simulink model "testmodel_1109"  (R2015b)
settings: Solver=FixedStepDiscrete  StartTime=0.0  StopTime=50  FixedStep=Ts  RelTol=1e-3
PreLoadFcn:
  | Ts_IO601 = 0.001;
InitFcn:
  | Ts_IO601 = 0.001;
  | Ts=0.004;
libraries: canmsglib x14, speedgoatlib_IO601 x9, slrtlib x9, simulink x3
settings Model: Creator=lab2  LastModifiedBy=1SMARTe
settings SolverCC: EnableConcurrentExecution=on
settings DataIOCC: SaveFormat=Array
settings OptimizationCC: BlockReduction=off  OptimizeBlockIOStorage=off  BufferReuse=off  GlobalBufferReuse=off  ExpressionFolding=off  LocalBlockOutputs=off
settings DebuggingCC: UnconnectedInputMsg=none  UnconnectedOutputMsg=none  UnconnectedLineMsg=none
settings HardwareCC: ProdBitPerPointer=32  ProdLargestAtomicFloat=None  ProdWordSize=32  ProdLongLongMode=on  ProdHWDeviceType=Generic->32-bit x86 compatible
settings RTWCC: SystemTargetFile=slrt.tlc  TemplateMakefile=slrt_default_tmf  Description=Simulink Real-Time  RTWCompilerOptimization=on
settings ConfigComp: CovModelRefEnable=Off

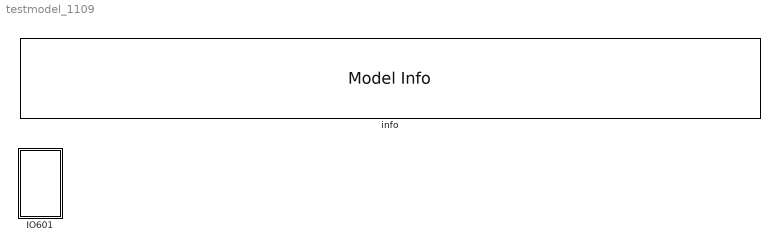
== system testmodel_1109 ==
  IO601 : Subsystem
  info : simulink/Model-Wide Utilities/Model Info  Frame=on  DisplayStringWithTags=|  HorizontalTextAlignment=Left  LeftAlignmentValue=0.02  SourceBlockDiagram=testmodel_1109  TagMaxNumber=20
      | SPEEDGOAT Simulink Real-Time  test model for Real-time target machine (SN2820)
      | prepared by Speedgoat with MATLAB R2015a
      | 
      | Build date: %<Created>

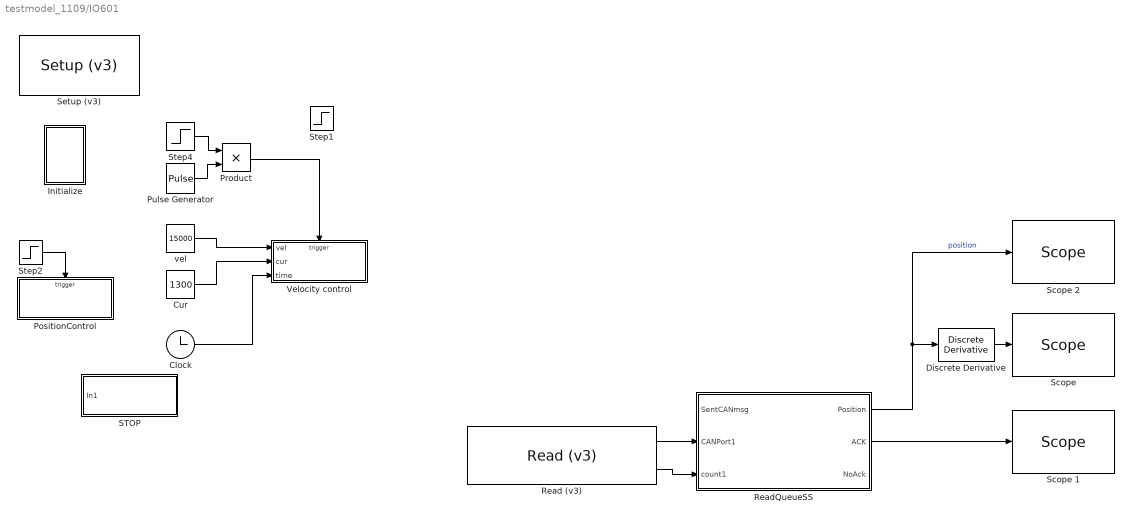
== system testmodel_1109/IO601 ==
  Clock : Clock
  Cur : Constant  Value=1300  OutMin=1100  OutMax=1500  OutDataTypeStr=uint32
  Discrete Derivative : simulink/Discrete/Discrete Derivative  gainval=1.0  ICPrevScaledInput=0.0  InputProcessing=Inherited  OutMin=[]  OutMax=[]  OutDataType=fixdt(1, 16)  OutScaling=2^-10  DoSatur=off
  Initialize : Subsystem
  "PositionControl " : Subsystem  TreatAsAtomicUnit=on
  Product : Product
  Pulse Generator : DiscretePulseGenerator  PulseType=Time based  Period=Ts*10  PulseWidth=10  PhaseDelay=10  SampleTime=Ts_IO601
  Read (v3) : speedgoatlib_IO601/Read (v3)  id=1  outputFormat=Vector of CAN_MESSAGE  port1=on  port2=off  depth1=37  depth2=4  sampletime=Ts  pciSlot=-1
  ReadQueueSS : Subsystem
  STOP : Subsystem  TreatAsAtomicUnit=on
  "Scope " : slrtlib/Displays and Logging/Scope   scopeno=3  scopetype=Target  autostart=on  viewmode=Graphical sliding  formatstr='%15.6f'  grid=on  ylimits=[0000,0000]  nosamples=50/Ts  noprepostsamples=0  interleave=1  triggermode=FreeRun  triggersignal=1  trigsignalfromport=off  triggerlevel=0.0  triggerslope=Either  triggerscope=1  triggersample=0  filename=data.dat  mode=Lazy  writesize=512  autorestart=off  dynamicfilemode=off  maxwritefilesize=512*1024^2
  Scope 1 : slrtlib/Displays and Logging/Scope   scopeno=12  scopetype=Target  autostart=on  viewmode=Numerical  formatstr='%15.6f'  grid=on  ylimits=[0000,0000]  nosamples=50/Ts  noprepostsamples=0  interleave=1  triggermode=FreeRun  triggersignal=1  trigsignalfromport=on  triggerlevel=0.0  triggerslope=Either  triggerscope=1  triggersample=0  filename=data.dat  mode=Lazy  writesize=512  autorestart=off  dynamicfilemode=off  maxwritefilesize=512*1024^2
  Scope 2 : slrtlib/Displays and Logging/Scope   scopeno=2  scopetype=Target  autostart=on  viewmode=Graphical sliding  formatstr='%15.6f'  grid=on  ylimits=[0000,0000]  nosamples=50/Ts  noprepostsamples=0  interleave=1  triggermode=FreeRun  triggersignal=1  trigsignalfromport=off  triggerlevel=0.0  triggerslope=Either  triggerscope=1  triggersample=0  filename=data.dat  mode=Lazy  writesize=512  autorestart=off  dynamicfilemode=off  maxwritefilesize=512*1024^2
  Setup (v3) : speedgoatlib_IO601/Setup (v3)  id=1  can1enable=on  can1bus=Highspeed  can1Baudrate=1 MBaud  can1UserBR=[1,1,5,2]  stdAcc1=[0,0,0,0]  extAcc1=[0,0,0,0]  can2enable=on  can2bus=Highspeed  can2Baudrate=1 MBaud  can2UserBR=[1,1,5,2]  stdAcc2=[0,0,0,0]  extAcc2=[0,0,0,0]  pciSlot=-1
  Step1 : Step  Time=10  SampleTime=Ts
  Step2 : Step  Time=25  SampleTime=Ts
  Step4 : Step  Time=14  Before=1  After=0  SampleTime=0
  Velocity control : Subsystem  TreatAsAtomicUnit=on
  "vel " : Constant  Value=15000  OutMin=0  OutMax=20000  OutDataTypeStr=uint32
  wires:
  Step4/1 -> Product/1
  Pulse Generator/1 -> Product/2
  ReadQueueSS/2(ACK) -> Scope 1/1
  Cur/1 -> Velocity control/2(cur)
  "vel "/1 -> Velocity control/1(vel)
  ReadQueueSS/1(Position) -> Discrete Derivative/1, Scope 2/1  "position"
  Discrete Derivative/1 -> "Scope "/1
  Read (v3)/1 -> ReadQueueSS/2(CANPort1)
  Read (v3)/2 -> ReadQueueSS/3(count1)
  Step2/1 -> "PositionControl "/Trigger
  Product/1 -> Velocity control/Trigger
  Clock/1 -> Velocity control/3(time)

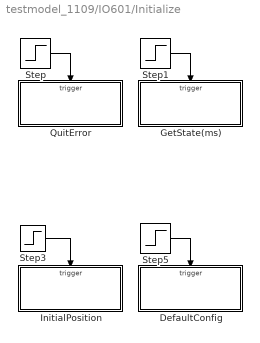
== system testmodel_1109/IO601/Initialize ==
  DefaultConfig : Subsystem  TreatAsAtomicUnit=on
  GetState(ms) : Subsystem  TreatAsAtomicUnit=on
  InitialPosition : Subsystem  TreatAsAtomicUnit=on
  QuitError : Subsystem  TreatAsAtomicUnit=on
  Step : Step  SampleTime=Ts
  Step1 : Step  Time=2  SampleTime=Ts
  Step3 : Step  Time=2  SampleTime=Ts
  Step5 : Step  Time=15  SampleTime=Ts
  wires:
  Step/1 -> QuitError/Trigger
  Step3/1 -> InitialPosition/Trigger
  Step5/1 -> DefaultConfig/Trigger
  Step1/1 -> GetState(ms)/Trigger

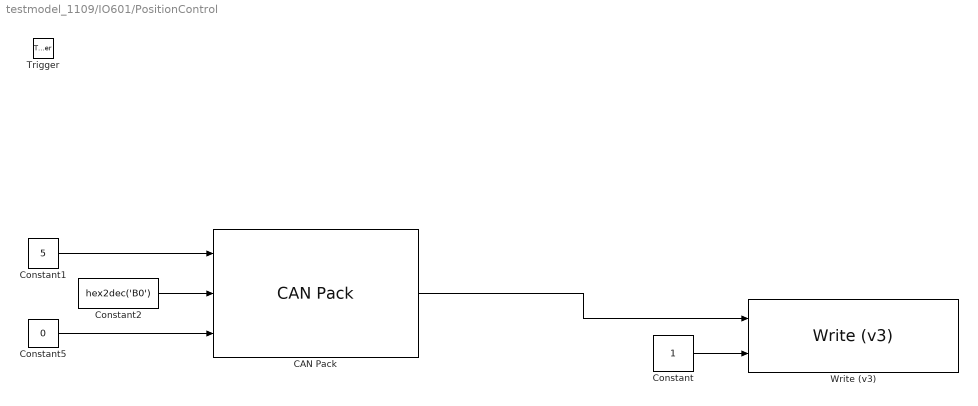
== system testmodel_1109/IO601/PositionControl  ==
  Trigger : TriggerPort
  CAN Pack : canmsglib/CAN Pack  MsgList=(none)  MsgName=Position Msg  MsgIDType=Standard (11-bit identifier)  MsgIdentifier=hex2dec('503')  MsgLength=6  SignalInfo=Signal1$0$8$1$2$1$0$1$0$-Inf$Inf$#Signal2$8$8$1$2$1$0$1$0$-Inf$Inf$#Signal3$16$32$1$1$1$0$1$0$-Inf$Inf$#  NSignals=3  StartBits=str2num('[int32(0);int32(8);int32(16)]')  SignalSizes=str2num('[int32(8);int32(8);int32(32)]')  ByteOrders=str2num('[int32(1);int32(1);int32(1)]')  DataTypes=str2num('[int32(2);int32(2);int32(1)]')  MultiplexTypes=str2num('[int32(1);int32(1);int32(1)]')  MultiplexValues=str2num('[double(0);double(0);double(0)]')  Factors=str2num('[double(1);double(1);double(1)]')  Offsets=str2num('[double(0);double(0);double(0)]')  Minimums=str2num('[double(-Inf);double(-Inf);double(-Inf)]')  Maximums=str2num('[double(Inf);double(Inf);double(Inf)]')  Remote=off
      settings: DataFormat=manually specified signals
  Constant : Constant
  Constant1 : Constant  Value=5
  Constant2 : Constant  Value=hex2dec('B0')
  Constant5 : Constant  Value=0
  Write (v3) : speedgoatlib_IO601/Write (v3)  Priority=1  id=1  sampletime=-1  pciSlot=-1  inputType=CAN_MESSAGE plus count  port=1  maxMsg=1  status=off  init=[]  term=[]
  wires:
  CAN Pack/1 -> Write (v3)/1
  Constant/1 -> Write (v3)/2
  Constant1/1 -> CAN Pack/1
  Constant2/1 -> CAN Pack/2
  Constant5/1 -> CAN Pack/3

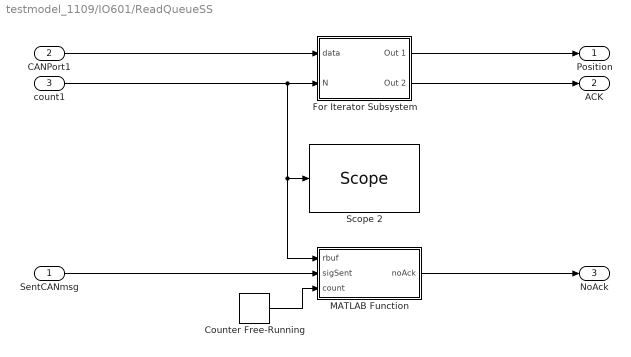
== system testmodel_1109/IO601/ReadQueueSS ==
  SentCANmsg : Inport
  CANPort1 : Inport  Port=2
  count1 : Inport  Port=3
  Counter Free-Running : simulink/Sources/Counter Free-Running  NumBits=2  tsamp=-1
  For Iterator Subsystem : Subsystem  TreatAsAtomicUnit=on
  MATLAB Function : MATLAB Function  TreatAsAtomicUnit=on
  Scope 2 : slrtlib/Displays and Logging/Scope   scopeno=21  scopetype=Target  autostart=on  viewmode=Numerical  formatstr='%15.6f'  grid=on  ylimits=[0,0]  nosamples=50/Ts  noprepostsamples=0  interleave=1  triggermode=FreeRun  triggersignal=1  trigsignalfromport=off  triggerlevel=0.0  triggerslope=Either  triggerscope=1  triggersample=0  filename=data.dat  mode=Lazy  writesize=512  autorestart=off  dynamicfilemode=off  maxwritefilesize=512*1024^2
  Position : Outport
  ACK : Outport  Port=2
  " NoAck" : Outport  Port=3
  wires:
  CANPort1/1 -> For Iterator Subsystem/1(data)
  count1/1 -> MATLAB Function/1(rbuf), Scope 2/1, For Iterator Subsystem/2(N)
  For Iterator Subsystem/1(Out 1) -> Position/1
  For Iterator Subsystem/2(Out 2) -> ACK/1
  Counter Free-Running/1 -> MATLAB Function/3(count)
  SentCANmsg/1 -> MATLAB Function/2(sigSent)
  MATLAB Function/1(noAck) -> " NoAck"/1

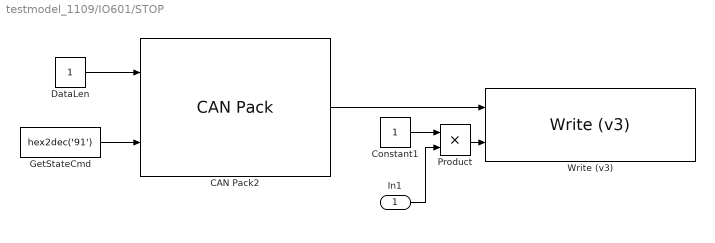
== system testmodel_1109/IO601/STOP ==
  In1 : Inport
  CAN Pack2 : canmsglib/CAN Pack  MsgList=(none)  MsgName=GetState  MsgIDType=Standard (11-bit identifier)  MsgIdentifier=hex2dec('503')  MsgLength=2  SignalInfo=Signal1$0$8$1$2$1$0$1$0$-Inf$Inf$#Signal2$8$8$1$2$1$0$1$0$-Inf$Inf$#  NSignals=2  StartBits=str2num('[int32(0);int32(8)]')  SignalSizes=str2num('[int32(8);int32(8)]')  ByteOrders=str2num('[int32(1);int32(1)]')  DataTypes=str2num('[int32(2);int32(2)]')  MultiplexTypes=str2num('[int32(1);int32(1)]')  MultiplexValues=str2num('[double(0);double(0)]')  Factors=str2num('[double(1);double(1)]')  Offsets=str2num('[double(0);double(0)]')  Minimums=str2num('[double(-Inf);double(-Inf)]')  Maximums=str2num('[double(Inf);double(Inf)]')  Remote=off
      settings: DataFormat=manually specified signals
  Constant1 : Constant
  DataLen : Constant
  GetStateCmd : Constant  Value=hex2dec('91')
  Product : Product
  Write (v3) : speedgoatlib_IO601/Write (v3)  Priority=1  id=1  sampletime=-1  pciSlot=-1  inputType=CAN_MESSAGE plus count  port=1  maxMsg=1  status=off  init=[]  term=[]
  wires:
  DataLen/1 -> CAN Pack2/1
  GetStateCmd/1 -> CAN Pack2/2
  CAN Pack2/1 -> Write (v3)/1
  Product/1 -> Write (v3)/2
  Constant1/1 -> Product/1
  In1/1 -> Product/2

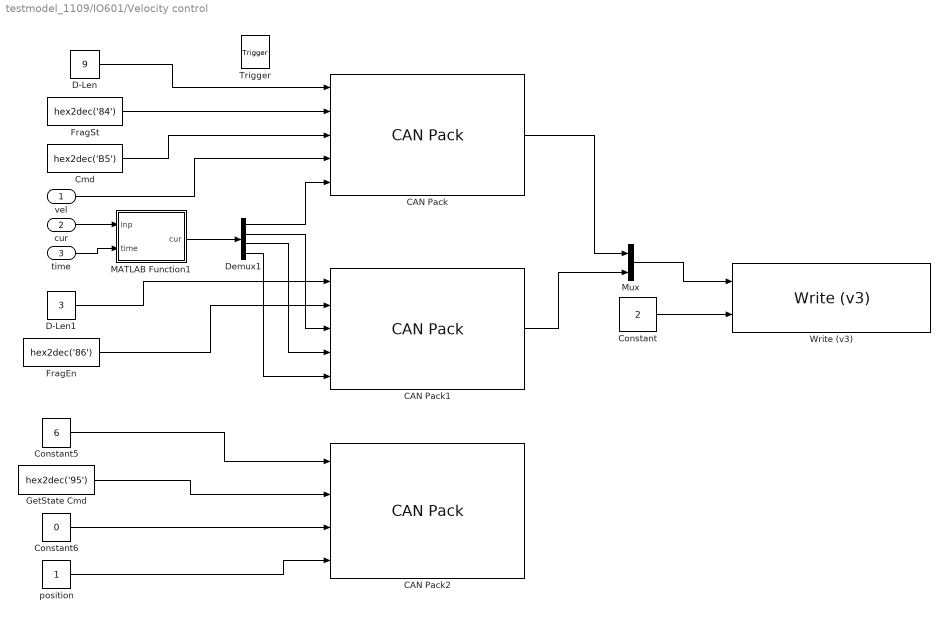
== system testmodel_1109/IO601/Velocity control ==
  vel : Inport
  cur : Inport  Port=2
  time : Inport  Port=3
  Trigger : TriggerPort
  CAN Pack : canmsglib/CAN Pack  MsgList=(none)  MsgName=Position Msg  MsgIDType=Standard (11-bit identifier)  MsgIdentifier=hex2dec('503')  MsgLength=8  SignalInfo=Signal1$0$8$1$2$1$0$1$0$-Inf$Inf$#Signal2$8$8$1$2$1$0$1$0$-Inf$Inf$#Signal3$16$8$1$2$1$0$1$0$-Inf$Inf$#Signal4$24$32$1$1$1$0$1$0$-Inf$Inf$#Signal5$56$8$1$2$1$0$1$0$-Inf$Inf$#  NSignals=5  StartBits=str2num('[int32(0);int32(8);int32(16);int32(24);int32(56)]')  SignalSizes=str2num('[int32(8);int32(8);int32(8);int32(32);int32(8)]')  ByteOrders=str2num('[int32(1);int32(1);int32(1);int32(1);int32(1)]')  DataTypes=str2num('[int32(2);int32(2);int32(2);int32(1);int32(2)]')  MultiplexTypes=str2num('[int32(1);int32(1);int32(1);int32(1);int32(1)]')  MultiplexValues=str2num('[double(0);double(0);double(0);double(0);double(0)]')  Factors=str2num('[double(1);double(1);double(1);double(1);double(1)]')  Offsets=str2num('[double(0);double(0);double(0);double(0);double(0)]')  Minimums=str2num('[double(-Inf);double(-Inf);double(-Inf);double(-Inf);double(-Inf)]')  Maximums=str2num('[double(Inf);double(Inf);double(Inf);double(Inf);double(Inf)]')  Remote=off
      settings: DataFormat=manually specified signals
  CAN Pack1 : canmsglib/CAN Pack  MsgList=(none)  MsgName=Position Msg  MsgIDType=Standard (11-bit identifier)  MsgIdentifier=hex2dec('503')  MsgLength=5  SignalInfo=Signal1$0$8$1$2$1$0$1$0$-Inf$Inf$#Signal2$8$8$1$2$1$0$1$0$-Inf$Inf$#Signal3$16$8$1$2$1$0$1$0$-Inf$Inf$#Signal4$24$8$1$2$1$0$1$0$-Inf$Inf$#Signal5$32$8$1$2$1$0$1$0$-Inf$Inf$#  NSignals=5  StartBits=str2num('[int32(0);int32(8);int32(16);int32(24);int32(32)]')  SignalSizes=str2num('[int32(8);int32(8);int32(8);int32(8);int32(8)]')  ByteOrders=str2num('[int32(1);int32(1);int32(1);int32(1);int32(1)]')  DataTypes=str2num('[int32(2);int32(2);int32(2);int32(2);int32(2)]')  MultiplexTypes=str2num('[int32(1);int32(1);int32(1);int32(1);int32(1)]')  MultiplexValues=str2num('[double(0);double(0);double(0);double(0);double(0)]')  Factors=str2num('[double(1);double(1);double(1);double(1);double(1)]')  Offsets=str2num('[double(0);double(0);double(0);double(0);double(0)]')  Minimums=str2num('[double(-Inf);double(-Inf);double(-Inf);double(-Inf);double(-Inf)]')  Maximums=str2num('[double(Inf);double(Inf);double(Inf);double(Inf);double(Inf)]')  Remote=off
      settings: DataFormat=manually specified signals
  CAN Pack2 : canmsglib/CAN Pack  MsgList=(none)  MsgName=GetState  MsgIDType=Standard (11-bit identifier)  MsgIdentifier=hex2dec('503')  MsgLength=7  SignalInfo=Signal1$0$8$1$2$1$0$1$0$-Inf$Inf$#Signal2$8$8$1$2$1$0$1$0$-Inf$Inf$#time$16$32$1$2$1$0$1$0$-Inf$Inf$#mode$48$8$1$2$1$0$1$0$-Inf$Inf$#  NSignals=4  StartBits=str2num('[int32(0);int32(8);int32(16);int32(48)]')  SignalSizes=str2num('[int32(8);int32(8);int32(32);int32(8)]')  ByteOrders=str2num('[int32(1);int32(1);int32(1);int32(1)]')  DataTypes=str2num('[int32(2);int32(2);int32(2);int32(2)]')  MultiplexTypes=str2num('[int32(1);int32(1);int32(1);int32(1)]')  MultiplexValues=str2num('[double(0);double(0);double(0);double(0)]')  Factors=str2num('[double(1);double(1);double(1);double(1)]')  Offsets=str2num('[double(0);double(0);double(0);double(0)]')  Minimums=str2num('[double(-Inf);double(-Inf);double(-Inf);double(-Inf)]')  Maximums=str2num('[double(Inf);double(Inf);double(Inf);double(Inf)]')  Remote=off
      settings: DataFormat=manually specified signals
  Cmd : Constant  Value=hex2dec('B5')
  Constant : Constant  Value=2
  Constant5 : Constant  Value=6
  Constant6 : Constant  Value=0
  D-Len : Constant  Value=9
  D-Len1 : Constant  Value=3
  Demux1 : Demux
  FragEn : Constant  Value=hex2dec('86')
  FragSt : Constant  Value=hex2dec('84')
  GetState Cmd : Constant  Value=hex2dec('95')
  MATLAB Function1 : MATLAB Function  TreatAsAtomicUnit=on
  Mux : Mux  Inputs=2
  Write (v3) : speedgoatlib_IO601/Write (v3)  Priority=1  id=1  sampletime=-1  pciSlot=-1  inputType=CAN_MESSAGE plus count  port=1  maxMsg=2  status=off  init=[]  term=[]
  position : Constant  OutDataTypeStr=uint8
  wires:
  Constant/1 -> Write (v3)/2
  D-Len/1 -> CAN Pack/1
  Cmd/1 -> CAN Pack/3
  Constant6/1 -> CAN Pack2/3
  Constant5/1 -> CAN Pack2/1
  GetState Cmd/1 -> CAN Pack2/2
  position/1 -> CAN Pack2/4
  CAN Pack/1 -> Mux/1
  Mux/1 -> Write (v3)/1
  FragSt/1 -> CAN Pack/2
  FragEn/1 -> CAN Pack1/2
  D-Len1/1 -> CAN Pack1/1
  CAN Pack1/1 -> Mux/2
  vel/1 -> CAN Pack/4
  MATLAB Function1/1(cur) -> Demux1/1
  Demux1/1 -> CAN Pack/5
  Demux1/2 -> CAN Pack1/3
  Demux1/3 -> CAN Pack1/4
  Demux1/4 -> CAN Pack1/5
  cur/1 -> MATLAB Function1/1(inp)
  time/1 -> MATLAB Function1/2(time)

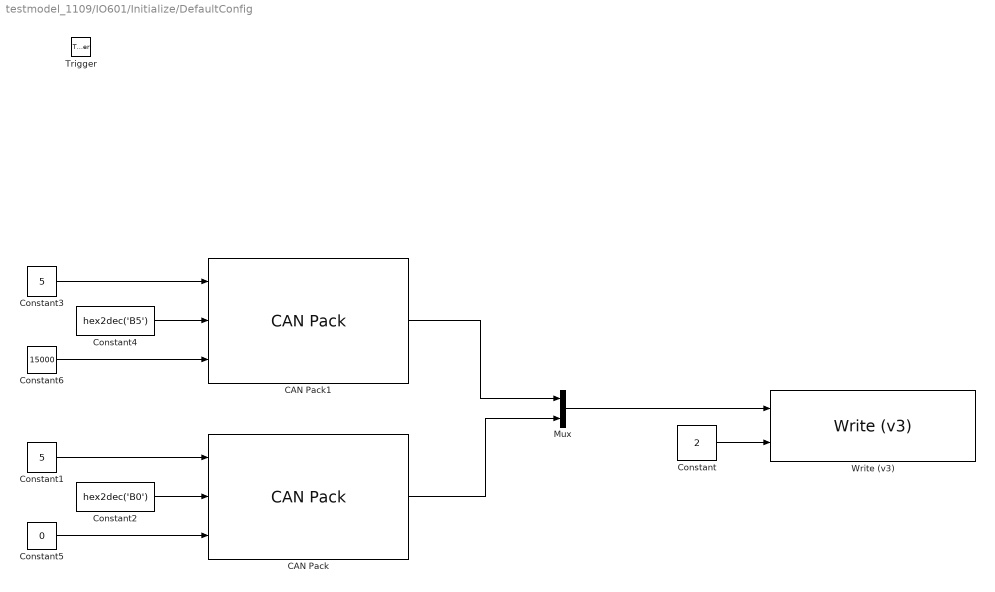
== system testmodel_1109/IO601/Initialize/DefaultConfig ==
  Trigger : TriggerPort
  CAN Pack : canmsglib/CAN Pack  MsgList=(none)  MsgName=Position Msg  MsgIDType=Standard (11-bit identifier)  MsgIdentifier=hex2dec('503')  MsgLength=6  SignalInfo=Signal1$0$8$1$2$1$0$1$0$-Inf$Inf$#Signal2$8$8$1$2$1$0$1$0$-Inf$Inf$#Signal3$16$32$1$1$1$0$1$0$-Inf$Inf$#  NSignals=3  StartBits=str2num('[int32(0);int32(8);int32(16)]')  SignalSizes=str2num('[int32(8);int32(8);int32(32)]')  ByteOrders=str2num('[int32(1);int32(1);int32(1)]')  DataTypes=str2num('[int32(2);int32(2);int32(1)]')  MultiplexTypes=str2num('[int32(1);int32(1);int32(1)]')  MultiplexValues=str2num('[double(0);double(0);double(0)]')  Factors=str2num('[double(1);double(1);double(1)]')  Offsets=str2num('[double(0);double(0);double(0)]')  Minimums=str2num('[double(-Inf);double(-Inf);double(-Inf)]')  Maximums=str2num('[double(Inf);double(Inf);double(Inf)]')  Remote=off
      settings: DataFormat=manually specified signals
  CAN Pack1 : canmsglib/CAN Pack  MsgList=(none)  MsgName=Position Msg  MsgIDType=Standard (11-bit identifier)  MsgIdentifier=hex2dec('503')  MsgLength=6  SignalInfo=Signal1$0$8$1$2$1$0$1$0$-Inf$Inf$#Signal2$8$8$1$2$1$0$1$0$-Inf$Inf$#Signal3$16$32$1$1$1$0$1$0$-Inf$Inf$#  NSignals=3  StartBits=str2num('[int32(0);int32(8);int32(16)]')  SignalSizes=str2num('[int32(8);int32(8);int32(32)]')  ByteOrders=str2num('[int32(1);int32(1);int32(1)]')  DataTypes=str2num('[int32(2);int32(2);int32(1)]')  MultiplexTypes=str2num('[int32(1);int32(1);int32(1)]')  MultiplexValues=str2num('[double(0);double(0);double(0)]')  Factors=str2num('[double(1);double(1);double(1)]')  Offsets=str2num('[double(0);double(0);double(0)]')  Minimums=str2num('[double(-Inf);double(-Inf);double(-Inf)]')  Maximums=str2num('[double(Inf);double(Inf);double(Inf)]')  Remote=off
      settings: DataFormat=manually specified signals
  Constant : Constant  Value=2
  Constant1 : Constant  Value=5
  Constant2 : Constant  Value=hex2dec('B0')
  Constant3 : Constant  Value=5
  Constant4 : Constant  Value=hex2dec('B5')
  Constant5 : Constant  Value=0
  Constant6 : Constant  Value=15000
  Mux : Mux  Inputs=2
  Write (v3) : speedgoatlib_IO601/Write (v3)  Priority=1  id=1  sampletime=-1  pciSlot=-1  inputType=CAN_MESSAGE plus count  port=1  maxMsg=2  status=off  init=[]  term=[]
  wires:
  CAN Pack/1 -> Mux/2
  Constant/1 -> Write (v3)/2
  Constant1/1 -> CAN Pack/1
  Constant2/1 -> CAN Pack/2
  Constant5/1 -> CAN Pack/3
  CAN Pack1/1 -> Mux/1
  Constant3/1 -> CAN Pack1/1
  Constant4/1 -> CAN Pack1/2
  Constant6/1 -> CAN Pack1/3
  Mux/1 -> Write (v3)/1

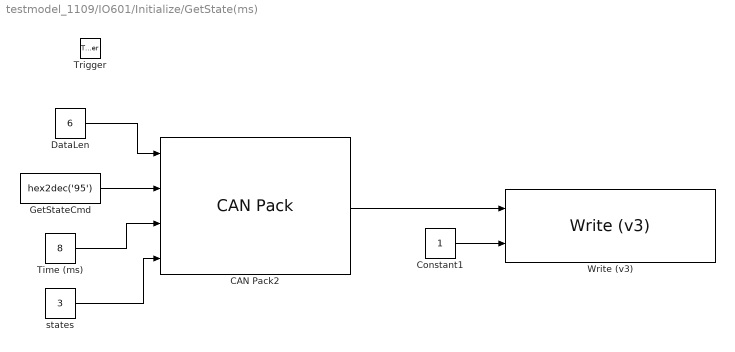
== system testmodel_1109/IO601/Initialize/GetState(ms) ==
  Trigger : TriggerPort
  CAN Pack2 : canmsglib/CAN Pack  MsgList=(none)  MsgName=GetState  MsgIDType=Standard (11-bit identifier)  MsgIdentifier=hex2dec('503')  MsgLength=7  SignalInfo=Signal1$0$8$1$2$1$0$1$0$-Inf$Inf$#Signal2$8$8$1$2$1$0$1$0$-Inf$Inf$#time$16$32$1$2$1$0$1$0$-Inf$Inf$#mode$48$8$1$2$1$0$1$0$-Inf$Inf$#  NSignals=4  StartBits=str2num('[int32(0);int32(8);int32(16);int32(48)]')  SignalSizes=str2num('[int32(8);int32(8);int32(32);int32(8)]')  ByteOrders=str2num('[int32(1);int32(1);int32(1);int32(1)]')  DataTypes=str2num('[int32(2);int32(2);int32(2);int32(2)]')  MultiplexTypes=str2num('[int32(1);int32(1);int32(1);int32(1)]')  MultiplexValues=str2num('[double(0);double(0);double(0);double(0)]')  Factors=str2num('[double(1);double(1);double(1);double(1)]')  Offsets=str2num('[double(0);double(0);double(0);double(0)]')  Minimums=str2num('[double(-Inf);double(-Inf);double(-Inf);double(-Inf)]')  Maximums=str2num('[double(Inf);double(Inf);double(Inf);double(Inf)]')  Remote=off
      settings: DataFormat=manually specified signals
  Constant1 : Constant
  DataLen : Constant  Value=6
  GetStateCmd : Constant  Value=hex2dec('95')
  Time (ms) : Constant  Value=8
  Write (v3) : speedgoatlib_IO601/Write (v3)  Priority=1  id=1  sampletime=-1  pciSlot=-1  inputType=CAN_MESSAGE plus count  port=1  maxMsg=1  status=off  init=[]  term=[]
  states : Constant  Value=3  OutDataTypeStr=uint8
  wires:
  Constant1/1 -> Write (v3)/2
  Time (ms)/1 -> CAN Pack2/3
  DataLen/1 -> CAN Pack2/1
  GetStateCmd/1 -> CAN Pack2/2
  CAN Pack2/1 -> Write (v3)/1
  states/1 -> CAN Pack2/4

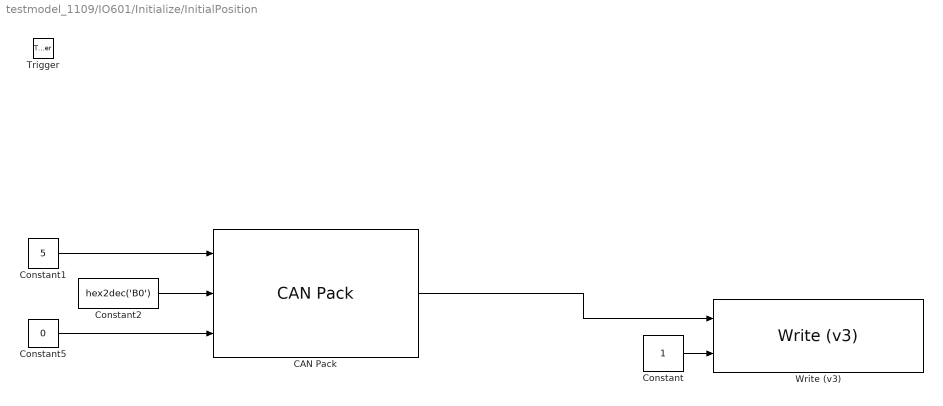
== system testmodel_1109/IO601/Initialize/InitialPosition ==
  Trigger : TriggerPort
  CAN Pack : canmsglib/CAN Pack  MsgList=(none)  MsgName=Position Msg  MsgIDType=Standard (11-bit identifier)  MsgIdentifier=1283  MsgLength=6  SignalInfo=Signal1$0$8$1$2$1$0$1$0$-Inf$Inf$#Signal2$8$8$1$2$1$0$1$0$-Inf$Inf$#Signal3$16$32$1$1$1$0$1$0$-Inf$Inf$#  NSignals=3  StartBits=str2num('[int32(0);int32(8);int32(16)]')  SignalSizes=str2num('[int32(8);int32(8);int32(32)]')  ByteOrders=str2num('[int32(1);int32(1);int32(1)]')  DataTypes=str2num('[int32(2);int32(2);int32(1)]')  MultiplexTypes=str2num('[int32(1);int32(1);int32(1)]')  MultiplexValues=str2num('[double(0);double(0);double(0)]')  Factors=str2num('[double(1);double(1);double(1)]')  Offsets=str2num('[double(0);double(0);double(0)]')  Minimums=str2num('[double(-Inf);double(-Inf);double(-Inf)]')  Maximums=str2num('[double(Inf);double(Inf);double(Inf)]')  Remote=off
      settings: DataFormat=manually specified signals
  Constant : Constant
  Constant1 : Constant  Value=5
  Constant2 : Constant  Value=hex2dec('B0')
  Constant5 : Constant  Value=0
  Write (v3) : speedgoatlib_IO601/Write (v3)  Priority=1  id=1  sampletime=-1  pciSlot=-1  inputType=CAN_MESSAGE plus count  port=1  maxMsg=1  status=off  init=[]  term=[]
  wires:
  CAN Pack/1 -> Write (v3)/1
  Constant/1 -> Write (v3)/2
  Constant1/1 -> CAN Pack/1
  Constant2/1 -> CAN Pack/2
  Constant5/1 -> CAN Pack/3

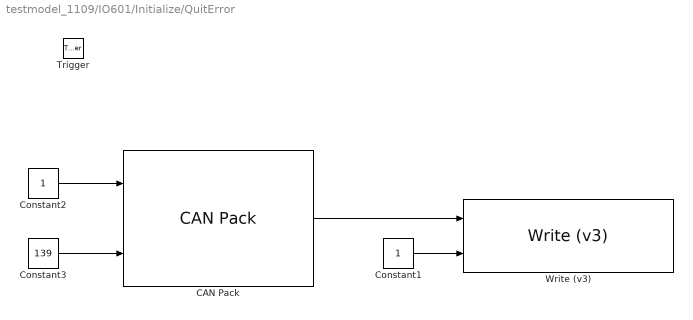
== system testmodel_1109/IO601/Initialize/QuitError ==
  Trigger : TriggerPort
  CAN Pack : canmsglib/CAN Pack  MsgList=(none)  MsgName=QuitError  MsgIDType=Standard (11-bit identifier)  MsgIdentifier=hex2dec('503')  MsgLength=2  SignalInfo=Signal1$0$8$1$2$1$0$1$0$-Inf$Inf$#Signal2$8$8$1$2$1$0$1$0$-Inf$Inf$#  NSignals=2  StartBits=str2num('[int32(0);int32(8)]')  SignalSizes=str2num('[int32(8);int32(8)]')  ByteOrders=str2num('[int32(1);int32(1)]')  DataTypes=str2num('[int32(2);int32(2)]')  MultiplexTypes=str2num('[int32(1);int32(1)]')  MultiplexValues=str2num('[double(0);double(0)]')  Factors=str2num('[double(1);double(1)]')  Offsets=str2num('[double(0);double(0)]')  Minimums=str2num('[double(-Inf);double(-Inf)]')  Maximums=str2num('[double(Inf);double(Inf)]')  Remote=off
      settings: DataFormat=manually specified signals
  Constant1 : Constant
  Constant2 : Constant
  Constant3 : Constant  Value=139
  Write (v3) : speedgoatlib_IO601/Write (v3)  Priority=1  id=1  sampletime=-1  pciSlot=-1  inputType=CAN_MESSAGE plus count  port=1  maxMsg=1  status=off  init=[]  term=[]
  wires:
  Constant3/1 -> CAN Pack/2
  Constant2/1 -> CAN Pack/1
  CAN Pack/1 -> Write (v3)/1
  Constant1/1 -> Write (v3)/2

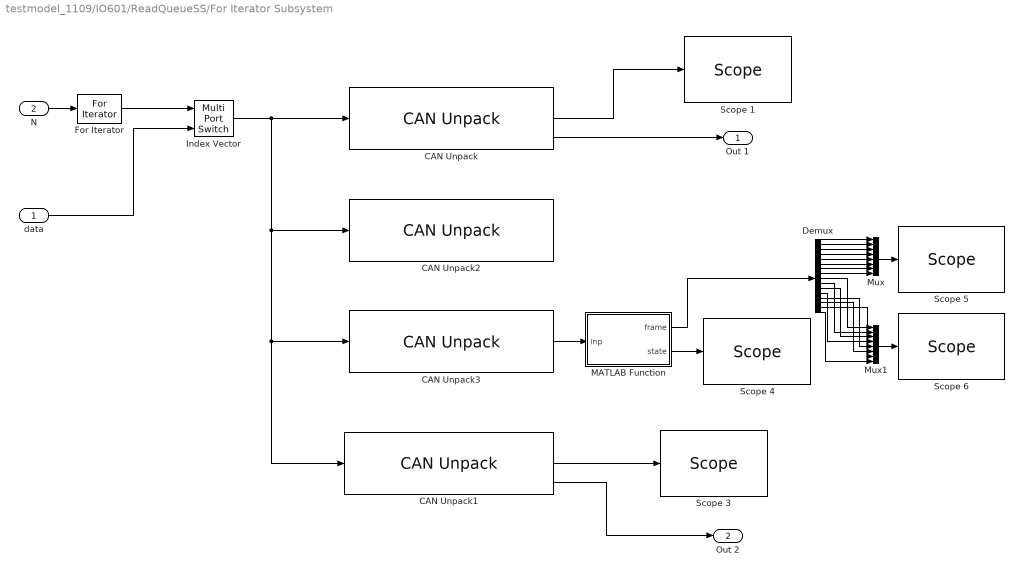
== system testmodel_1109/IO601/ReadQueueSS/For Iterator Subsystem ==
  data : Inport
  N : Inport  Port=2
  CAN Unpack : canmsglib/CAN Unpack  MsgList=(none)  MsgName=Message20  MsgIDType=Standard (11-bit identifier)  MsgIdentifier=hex2dec('703')  MsgLength=8  SignalInfo=DLen$0$8$1$2$1$0$1$0$-Inf$Inf$#Cmd$8$8$1$2$1$0$1$0$-Inf$Inf$#Position$16$32$1$1$1$0$1$0$-Inf$Inf$#  NSignals=3  IDPort=off  TimestampPort=off  ErrorPort=off  RemotePort=off  LengthPort=off  StatusPort=off  StartBits=str2num('[int32(0);int32(8);int32(16)]')  SignalSizes=str2num('[int32(8);int32(8);int32(32)]')  ByteOrders=str2num('[int32(1);int32(1);int32(1)]')  DataTypes=str2num('[int32(2);int32(2);int32(1)]')  MultiplexTypes=str2num('[int32(1);int32(1);int32(1)]')  MultiplexValues=str2num('[double(0);double(0);double(0)]')  Factors=str2num('[double(1);double(1);double(1)]')  Offsets=str2num('[double(0);double(0);double(0)]')  Minimums=str2num('[double(-Inf);double(-Inf);double(-Inf)]')  Maximums=str2num('[double(Inf);double(Inf);double(Inf)]')
  CAN Unpack1 : canmsglib/CAN Unpack  MsgList=(none)  MsgName=Message21  MsgIDType=Standard (11-bit identifier)  MsgIdentifier=hex2dec('703')  MsgLength=4  SignalInfo=DLen$0$8$1$2$1$0$1$0$-Inf$Inf$#Cmd$8$8$1$2$1$0$1$0$-Inf$Inf$#Param$16$16$1$1$1$0$1$0$-Inf$Inf$#  NSignals=3  IDPort=off  TimestampPort=off  ErrorPort=off  RemotePort=off  LengthPort=off  StatusPort=off  StartBits=str2num('[int32(0);int32(8);int32(16)]')  SignalSizes=str2num('[int32(8);int32(8);int32(16)]')  ByteOrders=str2num('[int32(1);int32(1);int32(1)]')  DataTypes=str2num('[int32(2);int32(2);int32(1)]')  MultiplexTypes=str2num('[int32(1);int32(1);int32(1)]')  MultiplexValues=str2num('[double(0);double(0);double(0)]')  Factors=str2num('[double(1);double(1);double(1)]')  Offsets=str2num('[double(0);double(0);double(0)]')  Minimums=str2num('[double(-Inf);double(-Inf);double(-Inf)]')  Maximums=str2num('[double(Inf);double(Inf);double(Inf)]')
  CAN Unpack2 : canmsglib/CAN Unpack  MsgList=(none)  MsgName=CANGSraw  MsgIDType=Standard (11-bit identifier)  MsgIdentifier=hex2dec('703')  MsgLength=8  SignalInfo=DLen$0$8$1$2$1$0$1$0$-Inf$Inf$#Cmd$8$8$1$2$1$0$1$0$-Inf$Inf$#Position$16$32$1$1$1$0$1$0$-Inf$Inf$#  NSignals=3  IDPort=off  TimestampPort=off  ErrorPort=off  RemotePort=off  LengthPort=off  StatusPort=off  StartBits=str2num('[int32(0);int32(8);int32(16)]')  SignalSizes=str2num('[int32(8);int32(8);int32(32)]')  ByteOrders=str2num('[int32(1);int32(1);int32(1)]')  DataTypes=str2num('[int32(2);int32(2);int32(1)]')  MultiplexTypes=str2num('[int32(1);int32(1);int32(1)]')  MultiplexValues=str2num('[double(0);double(0);double(0)]')  Factors=str2num('[double(1);double(1);double(1)]')  Offsets=str2num('[double(0);double(0);double(0)]')  Minimums=str2num('[double(-Inf);double(-Inf);double(-Inf)]')  Maximums=str2num('[double(Inf);double(Inf);double(Inf)]')
      settings: DataFormat=raw data
  CAN Unpack3 : canmsglib/CAN Unpack  MsgList=(none)  MsgName=CANGSraw2  MsgIDType=Standard (11-bit identifier)  MsgIdentifier=hex2dec('703')  MsgLength=8  SignalInfo=DLen$0$8$1$2$1$0$1$0$-Inf$Inf$#Cmd$8$8$1$2$1$0$1$0$-Inf$Inf$#Position$16$32$1$1$1$0$1$0$-Inf$Inf$#  NSignals=3  IDPort=off  TimestampPort=off  ErrorPort=off  RemotePort=off  LengthPort=off  StatusPort=off  StartBits=str2num('[int32(0);int32(8);int32(16)]')  SignalSizes=str2num('[int32(8);int32(8);int32(32)]')  ByteOrders=str2num('[int32(1);int32(1);int32(1)]')  DataTypes=str2num('[int32(2);int32(2);int32(1)]')  MultiplexTypes=str2num('[int32(1);int32(1);int32(1)]')  MultiplexValues=str2num('[double(0);double(0);double(0)]')  Factors=str2num('[double(1);double(1);double(1)]')  Offsets=str2num('[double(0);double(0);double(0)]')  Minimums=str2num('[double(-Inf);double(-Inf);double(-Inf)]')  Maximums=str2num('[double(Inf);double(Inf);double(Inf)]')
      settings: DataFormat=raw data
  Demux : Demux  Outputs=16
  For Iterator : ForIterator  IterationSource=external  IterationLimit=20  IterationVariableDataType=int8
  Index Vector : MultiPortSwitch  Inputs=1
  MATLAB Function : MATLAB Function  TreatAsAtomicUnit=on
  Mux : Mux  Inputs=8
  Mux1 : Mux  Inputs=8
  Scope 1 : slrtlib/Displays and Logging/Scope   scopeno=1  scopetype=Target  autostart=on  viewmode=Numerical  formatstr='%15.6f'  grid=on  ylimits=[-90000,90000]  nosamples=50/Ts  noprepostsamples=0  interleave=1  triggermode=FreeRun  triggersignal=1  trigsignalfromport=off  triggerlevel=0.0  triggerslope=Either  triggerscope=1  triggersample=0  filename=data.dat  mode=Lazy  writesize=512  autorestart=off  dynamicfilemode=off  maxwritefilesize=512*1024^2
  Scope 3 : slrtlib/Displays and Logging/Scope   scopeno=10  scopetype=Target  autostart=on  viewmode=Numerical  formatstr='%15.6f'  grid=on  ylimits=[-90000,90000]  nosamples=50/Ts  noprepostsamples=0  interleave=1  triggermode=FreeRun  triggersignal=1  trigsignalfromport=off  triggerlevel=0.0  triggerslope=Either  triggerscope=1  triggersample=0  filename=data.dat  mode=Lazy  writesize=512  autorestart=off  dynamicfilemode=off  maxwritefilesize=512*1024^2
  Scope 4 : slrtlib/Displays and Logging/Scope   scopeno=31  scopetype=Target  autostart=on  viewmode=Graphical sliding  formatstr='%15.6f'  grid=on  ylimits=[-90000,90000]  nosamples=50/Ts  noprepostsamples=0  interleave=1  triggermode=FreeRun  triggersignal=1  trigsignalfromport=off  triggerlevel=0.0  triggerslope=Either  triggerscope=1  triggersample=0  filename=data.dat  mode=Lazy  writesize=512  autorestart=off  dynamicfilemode=off  maxwritefilesize=512*1024^2
  Scope 5 : slrtlib/Displays and Logging/Scope   scopeno=33  scopetype=Target  autostart=on  viewmode=Numerical  formatstr='%15.6f'  grid=on  ylimits=[-90000,90000]  nosamples=50/Ts  noprepostsamples=0  interleave=1  triggermode=FreeRun  triggersignal=1  trigsignalfromport=off  triggerlevel=0.0  triggerslope=Either  triggerscope=1  triggersample=0  filename=data.dat  mode=Lazy  writesize=512  autorestart=off  dynamicfilemode=off  maxwritefilesize=512*1024^2
  Scope 6 : slrtlib/Displays and Logging/Scope   scopeno=34  scopetype=Target  autostart=on  viewmode=Numerical  formatstr='%15.6f'  grid=on  ylimits=[-90000,90000]  nosamples=50/Ts  noprepostsamples=0  interleave=1  triggermode=FreeRun  triggersignal=1  trigsignalfromport=off  triggerlevel=0.0  triggerslope=Either  triggerscope=1  triggersample=0  filename=data.dat  mode=Lazy  writesize=512  autorestart=off  dynamicfilemode=off  maxwritefilesize=512*1024^2
  Out 1 : Outport
  Out 2 : Outport  Port=2
  wires:
  For Iterator/1 -> Index Vector/1
  data/1 -> Index Vector/2
  N/1 -> For Iterator/1
  CAN Unpack/2 -> Scope 1/1
  CAN Unpack/3 -> Out 1/1
  CAN Unpack1/3 -> Out 2/1
  CAN Unpack1/2 -> Scope 3/1
  Index Vector/1 -> CAN Unpack2/1, CAN Unpack3/1, CAN Unpack1/1, CAN Unpack/1
  CAN Unpack3/1 -> MATLAB Function/1(inp)
  MATLAB Function/2(state) -> Scope 4/1
  Demux/7 -> Mux/7
  Demux/8 -> Mux/8
  Demux/6 -> Mux/6
  Demux/3 -> Mux/3
  Demux/5 -> Mux/5
  Demux/4 -> Mux/4
  Demux/1 -> Mux/1
  Demux/2 -> Mux/2
  Mux/1 -> Scope 5/1
  Mux1/1 -> Scope 6/1
  Demux/9 -> Mux1/1
  Demux/10 -> Mux1/2
  Demux/11 -> Mux1/3
  Demux/12 -> Mux1/4
  Demux/13 -> Mux1/5
  Demux/14 -> Mux1/6
  Demux/15 -> Mux1/7
  Demux/16 -> Mux1/8
  MATLAB Function/1(frame) -> Demux/1

== matlab function testmodel_1109/IO601/ReadQueueSS/MATLAB Function ==
  data: rbuf input; sigSent input; noAck output; count input
function noAck = checkACK(rbuf, sigSent, count)
%#codegen
noAck = 0;
if sigSent
    if rbuf == 0 && count == 4
        noAck = 1;
    else
        noAck = 0;
    end
end
end

== matlab function testmodel_1109/IO601/Velocity control/MATLAB Function1 ==
  data: cur output uint8 size=[1 4]; inp input uint32; time input
function cur   = fcn(inp, time)
%#codegen

c = (inp + 100*sin(2*pi*100/time));
cur = typecast((c), 'uint8');

% if cp > 0
%     vel = 90000;
% else
%     vel = -90000;
% end
end

== matlab function testmodel_1109/IO601/ReadQueueSS/For Iterator Subsystem/MATLAB Function ==
  data: inp input; frame output; state output int32 size=[1 3]
function [frame,state]  = decrypt_gs(inp)
%#codegen

persistent stitched;
persistent pos;
persistent vel;
persistent cur;

if isempty(stitched)
   stitched = zeros(1,16);
   pos = zeros(1,4);
   vel = zeros(1,4);
   cur = zeros(1,4);
end

compare = [7 inp(1) stitched(1)];
stitched(1) = max(compare);
if (inp(3)==hex2dec('95')) || (stitched(2)==hex2dec('95'))
    if inp(2) == hex2dec('84')            %first fragment
        stitched(2:7) = inp(3:8);             %cmd 4pos 1vel
        pos(1:4) = inp(4:7);
        vel(1) = int8(inp(8))
    elseif inp(2) == hex2dec('85')        %middle fragment
        stitched(8:13) = inp(3:8);             %3vel 3cur
        vel(2:4) = inp(3:5);
        cur(1:3) = inp(6:8)
    elseif inp(2) == hex2dec('86')        %last fragment
        if stitched(1) > 13
            stitched(14:16) = inp(3:5);        %1cur 2err
            cur(4) = inp(3);
        else
            stitched(8:12) = inp(3:7);         %3vel 2err
            vel(2:4) = inp(3:5)
        end

    elseif inp(2) == hex2dec('95')        %no fragment
        stitched(2:8) = inp(2:8);
        pos(1:4) = inp(3:6);
    end
end
frame = (stitched);

pos1 = typecast( uint8(pos) , 'int32');
vel1 = typecast( uint8(vel) , 'int32');
cur1 = typecast( uint8(cur) , 'int32');

pos1 = pos1(1); vel1 = vel1(1); cur1 = cur1(1);
state = [pos1 vel1 cur1];

% vel = 0;
% pos1 = [0 0 0 0];
% vel1 = [0 0 0 0];
% if u(2) == hex2dec('84')            %first fragment
%     pos1 = u(4:7); vel1(1) = u(8);
% elseif u(2) == hex2dec('85')        %middle fragment
%     
% elseif u(2) == hex2dec('86')        %last fragment
%     vel1(2:4) = u(3:5);
% elseif u(2) == hex2dec('95')        %no fragment
%     pos1 = u(3:6);
% end
% 
% pos = typecast(uint8(pos1), 'uint32');
% vel = typecast(uint8(vel1), 'uint32');
% 

end
